simulink model "EHB_MOTOR"  (R2023b)
settings: Solver=FixedStepDiscrete  StartTime=0.0  StopTime=inf  FixedStep=0.0001  RelTol=1e-3  EnableMultiTasking=on
undefined symbols (not defined in the file): CAN_EHB_VCU0x125, CAN_EHB_VCU0x126, CAN_id0x120_Data, Cos_Table, Cos_Table1, EHB_DTC_status, R, Sin_BreakPoint, Sin_BreakPoint1, Sin_Table, Sin_Table1, T
libraries: simulink x30
(part 4 of 9)

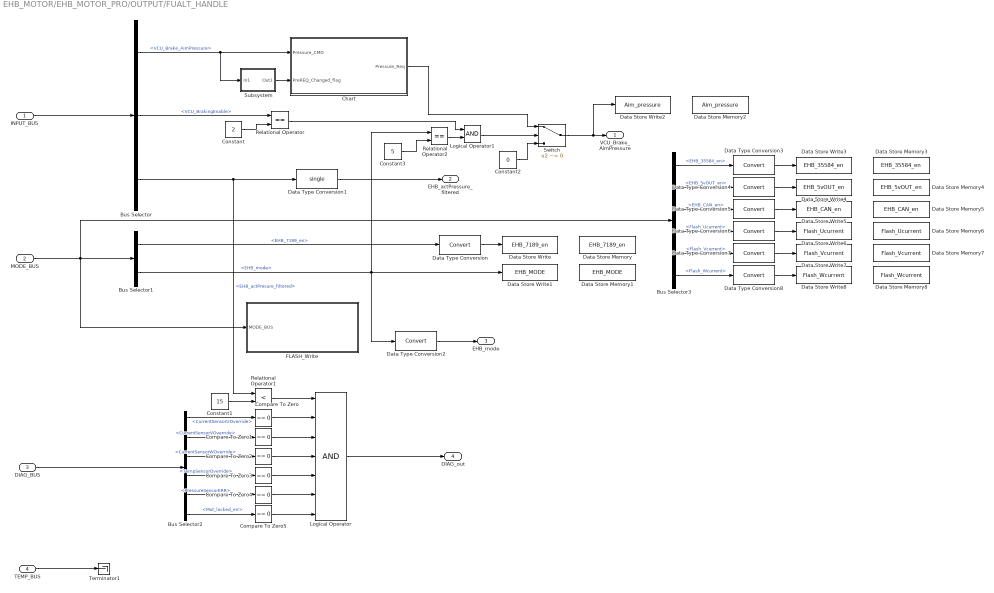
== system EHB_MOTOR/EHB_MOTOR_PRO/OUTPUT/FUALT_HANDLE ==
  INPUT_BUS : Inport
  MODE_BUS : Inport  Port=2
  DIAG_BUS : Inport  Port=3
  TEMP_BUS : Inport  Port=4
  Bus Selector : BusSelector  OutputSignals=CAN_BUS.VCU_Brake_AimPressure,CAN_BUS.VCU_BrakingEnable,AI_BUS.EHB_actPresure_filtered
  Bus Selector1 : BusSelector  OutputSignals=EHB_7189_en,EHB_mode
  Bus Selector2 : BusSelector  OutputSignals=CurrentSensorUOverride,CurrentSensorVOverride,CurrentSensorWOverride,TempSensorOverride,PressureSensorERR,Mot_locked_err
  Bus Selector3 : BusSelector  OutputSignals=EHB_35584_en,EHB_5vOUT_en,EHB_CAN_en,Flash_Ucurrent,Flash_Vcurrent,Flash_Wcurrent
  Chart : Stateflow chart  TreatAsAtomicUnit=on
  Compare To Zero{,1..5} (6 alike) : simulink/Logic and Bit Operations/Compare To Zero  relop===  OutDataTypeStr=boolean
  Constant : Constant  Value=2  OutDataTypeStr=Inherit: Inherit via back propagation
  Constant1 : Constant  Value=15
  Constant2 : Constant  Value=0  OutDataTypeStr=single
  Constant3 : Constant  Value=5  OutDataTypeStr=Inherit: Inherit via back propagation
  Data Store Memory : DataStoreMemory  DataStoreName=EHB_7189_en  ReadBeforeWriteMsg=warning  WriteAfterWriteMsg=warning  WriteAfterReadMsg=warning  ShowAdditionalParam=off  OutDataTypeStr=uint8
  Data Store Memory1 : DataStoreMemory  DataStoreName=EHB_MODE  ReadBeforeWriteMsg=warning  WriteAfterWriteMsg=warning  WriteAfterReadMsg=warning  ShowAdditionalParam=off  OutDataTypeStr=uint8
  Data Store Memory2 : DataStoreMemory  DataStoreName=Aim_pressure  ReadBeforeWriteMsg=warning  WriteAfterWriteMsg=warning  WriteAfterReadMsg=warning  ShowAdditionalParam=off  OutDataTypeStr=single
  Data Store Memory3 : DataStoreMemory  DataStoreName=EHB_35584_en  ReadBeforeWriteMsg=warning  WriteAfterWriteMsg=warning  WriteAfterReadMsg=warning  ShowAdditionalParam=off  OutDataTypeStr=uint8
  Data Store Memory4 : DataStoreMemory  DataStoreName=EHB_5vOUT_en  ReadBeforeWriteMsg=warning  WriteAfterWriteMsg=warning  WriteAfterReadMsg=warning  ShowAdditionalParam=off  OutDataTypeStr=uint8
  Data Store Memory5 : DataStoreMemory  DataStoreName=EHB_CAN_en  ReadBeforeWriteMsg=warning  WriteAfterWriteMsg=warning  WriteAfterReadMsg=warning  ShowAdditionalParam=off  OutDataTypeStr=uint8
  Data Store Memory6 : DataStoreMemory  DataStoreName=Flash_Ucurrent  ReadBeforeWriteMsg=warning  WriteAfterWriteMsg=warning  WriteAfterReadMsg=warning  ShowAdditionalParam=off  OutDataTypeStr=uint16
  Data Store Memory7 : DataStoreMemory  DataStoreName=Flash_Vcurrent  ReadBeforeWriteMsg=warning  WriteAfterWriteMsg=warning  WriteAfterReadMsg=warning  ShowAdditionalParam=off  OutDataTypeStr=uint16
  Data Store Memory8 : DataStoreMemory  DataStoreName=Flash_Wcurrent  ReadBeforeWriteMsg=warning  WriteAfterWriteMsg=warning  WriteAfterReadMsg=warning  ShowAdditionalParam=off  OutDataTypeStr=uint16
  Data Store Write : DataStoreWrite  DataStoreName=EHB_7189_en  DataStoreElements=EHB_7189_en  IndexOptions=Index vector (dialog)  Indices=1  OutputSizes=1
  Data Store Write1 : DataStoreWrite  DataStoreName=EHB_MODE  DataStoreElements=EHB_MODE  IndexOptions=Index vector (dialog)  Indices=1  OutputSizes=1
  Data Store Write2 : DataStoreWrite  DataStoreName=Aim_pressure  DataStoreElements=Aim_pressure  IndexOptions=Index vector (dialog)  Indices=1  OutputSizes=1
  Data Store Write3 : DataStoreWrite  DataStoreName=EHB_35584_en  DataStoreElements=EHB_35584_en  IndexOptions=Index vector (dialog)  Indices=1  OutputSizes=1
  Data Store Write4 : DataStoreWrite  DataStoreName=EHB_5vOUT_en  DataStoreElements=EHB_5vOUT_en  IndexOptions=Index vector (dialog)  Indices=1  OutputSizes=1
  Data Store Write5 : DataStoreWrite  DataStoreName=EHB_CAN_en  DataStoreElements=EHB_CAN_en  IndexOptions=Index vector (dialog)  Indices=1  OutputSizes=1
  Data Store Write6 : DataStoreWrite  DataStoreName=Flash_Ucurrent  DataStoreElements=Flash_Ucurrent  IndexOptions=Index vector (dialog)  Indices=1  OutputSizes=1
  Data Store Write7 : DataStoreWrite  DataStoreName=Flash_Vcurrent  DataStoreElements=Flash_Vcurrent  IndexOptions=Index vector (dialog)  Indices=1  OutputSizes=1
  Data Store Write8 : DataStoreWrite  DataStoreName=Flash_Wcurrent  DataStoreElements=Flash_Wcurrent  IndexOptions=Index vector (dialog)  Indices=1  OutputSizes=1
  Data Type Conversion{,2..8} (8 alike) : DataTypeConversion  SaturateOnIntegerOverflow=off  RndMeth=Floor
  Data Type Conversion1 : DataTypeConversion  OutDataTypeStr=single  SaturateOnIntegerOverflow=off  RndMeth=Floor
  FLASH_Write : Subsystem
  Logical Operator : Logic  Inputs=7  AllPortsSameDT=off  OutDataTypeStr=boolean
  Logical Operator1 : Logic  AllPortsSameDT=off  OutDataTypeStr=boolean
  Relational Operator : RelationalOperator  Operator===  OutDataTypeStr=boolean  RndMeth=Simplest  InputSameDT=off
  Relational Operator1 : RelationalOperator  Operator=<  OutDataTypeStr=boolean  RndMeth=Simplest  InputSameDT=off
  Relational Operator2 : RelationalOperator  Operator===  OutDataTypeStr=boolean  RndMeth=Simplest  InputSameDT=off
  Subsystem : Subsystem
  Switch : Switch  Criteria=u2 ~= 0  SaturateOnIntegerOverflow=off  InputSameDT=off
  Terminator1 : Terminator
  VCU_Brake_AimPressure : Outport  VectorParamsAs1DForOutWhenUnconnected=off
  EHB_actPressure_filtered : Outport  Port=2  VectorParamsAs1DForOutWhenUnconnected=off
  EHB_mode : Outport  Port=3  VectorParamsAs1DForOutWhenUnconnected=off
  DIAG_out : Outport  Port=4  VectorParamsAs1DForOutWhenUnconnected=off
  wires:
  INPUT_BUS/1 -> Bus Selector/1
  Bus Selector/3 -> Data Type Conversion1/1, Relational Operator1/1  "<EHB_actPresure_filtered>"
  TEMP_BUS/1 -> Terminator1/1
  MODE_BUS/1 -> Bus Selector1/1, FLASH_Write/1(MODE_BUS), Bus Selector3/1
  Bus Selector1/1 -> Data Type Conversion/1  "<EHB_7189_en>"
  Data Type Conversion/1 -> Data Store Write/1
  Bus Selector/1 -> Chart/1(Pressure_CMD), Subsystem/1(In1)  "<VCU_Brake_AimPressure>"
  Bus Selector/2 -> Relational Operator/1  "<VCU_BrakingEnable>"
  Constant/1 -> Relational Operator/2
  Relational Operator/1 -> Logical Operator1/1
  Switch/1 -> VCU_Brake_AimPressure/1, Data Store Write2/1
  Constant2/1 -> Switch/3
  Subsystem/1(Out1) -> Chart/2(PreREQ_Changed_flag)
  Chart/1(Pressure_Req) -> Switch/1
  Bus Selector2/4 -> Compare To Zero3/1  "<TempSensorOverride>"
  Bus Selector2/1 -> Compare To Zero/1  "<CurrentSensorUOverride>"
  Compare To Zero/1 -> Logical Operator/2
  Bus Selector2/2 -> Compare To Zero1/1  "<CurrentSensorVOverride>"
  Compare To Zero1/1 -> Logical Operator/3
  Compare To Zero2/1 -> Logical Operator/4
  Compare To Zero3/1 -> Logical Operator/5
  DIAG_BUS/1 -> Bus Selector2/1
  Bus Selector2/3 -> Compare To Zero2/1  "<CurrentSensorWOverride>"
  Logical Operator/1 -> DIAG_out/1
  Constant1/1 -> Relational Operator1/2
  Relational Operator1/1 -> Logical Operator/1
  Bus Selector1/2 -> Data Store Write1/1, Relational Operator2/1, Data Type Conversion2/1  "<EHB_mode>"
  Compare To Zero4/1 -> Logical Operator/6
  Bus Selector2/5 -> Compare To Zero4/1  "<PressureSensorERR>"
  Data Type Conversion1/1 -> EHB_actPressure_filtered/1
  Compare To Zero5/1 -> Logical Operator/7
  Bus Selector2/6 -> Compare To Zero5/1  "<Mot_locked_err>"
  Constant3/1 -> Relational Operator2/2
  Relational Operator2/1 -> Logical Operator1/2
  Logical Operator1/1 -> Switch/2
  Data Type Conversion2/1 -> EHB_mode/1
  Bus Selector3/1 -> Data Type Conversion3/1  "<EHB_35584_en>"
  Data Type Conversion3/1 -> Data Store Write3/1
  Bus Selector3/2 -> Data Type Conversion4/1  "<EHB_5vOUT_en>"
  Data Type Conversion4/1 -> Data Store Write4/1
  Data Type Conversion5/1 -> Data Store Write5/1
  Data Type Conversion6/1 -> Data Store Write6/1
  Bus Selector3/3 -> Data Type Conversion5/1  "<EHB_CAN_en>"
  Bus Selector3/4 -> Data Type Conversion6/1  "<Flash_Ucurrent>"
  Data Type Conversion7/1 -> Data Store Write7/1
  Data Type Conversion8/1 -> Data Store Write8/1
  Bus Selector3/5 -> Data Type Conversion7/1  "<Flash_Vcurrent>"
  Bus Selector3/6 -> Data Type Conversion8/1  "<Flash_Wcurrent>"

== system EHB_MOTOR/EHB_MOTOR_PRO/Pressure_closed/LOWPASS ==
  In1 : Inport
  Add : Sum
  Add1 : Sum  Inputs=+-
  Constant : Constant  Value=0.5  OutDataTypeStr=single
  Constant1 : Constant  OutDataTypeStr=single
  Multiply : Product
  Multiply1 : Product
  Unit Delay : UnitDelay  SampleTime=-1  HasFrameUpgradeWarning=on
  Out1 : Outport  VectorParamsAs1DForOutWhenUnconnected=off
  wires:
  In1/1 -> Multiply/1
  Multiply/1 -> Add/1
  Add/1 -> Unit Delay/1, Out1/1
  Constant/1 -> Add1/2, Multiply/2
  Constant1/1 -> Add1/1
  Add1/1 -> Multiply1/1
  Multiply1/1 -> Add/2
  Unit Delay/1 -> Multiply1/2

== system EHB_MOTOR/EHB_MOTOR_PRO/Speed_closed/Accuracy_Ctrl ==
  Pressure_Cmplt : Inport
  errSpd : Inport  Port=2
  SPDpterm_in : Inport  Port=3
  EHB_Initiate : Inport  Port=4
  Abs : Abs  SaturateOnIntegerOverflow=off
  Constant : Constant  Value=15  OutDataTypeStr=single
  Constant1 : Constant  Value=0  OutDataTypeStr=single
  Logical Operator : Logic  Operator=OR  Inputs=3  AllPortsSameDT=off  OutDataTypeStr=boolean
  Relational Operator : RelationalOperator  Operator=<=  OutDataTypeStr=boolean  RndMeth=Simplest  InputSameDT=off
  Switch : Switch  Criteria=u2 ~= 0  SaturateOnIntegerOverflow=off  InputSameDT=off
  SPDpterm_out : Outport  VectorParamsAs1DForOutWhenUnconnected=off
  wires:
  errSpd/1 -> Abs/1
  Abs/1 -> Relational Operator/1
  Constant/1 -> Relational Operator/2
  Switch/1 -> SPDpterm_out/1
  Constant1/1 -> Switch/1
  SPDpterm_in/1 -> Switch/3
  Relational Operator/1 -> Logical Operator/2
  Pressure_Cmplt/1 -> Logical Operator/1
  Logical Operator/1 -> Switch/2
  EHB_Initiate/1 -> Logical Operator/3

== system EHB_MOTOR/EHB_MOTOR_PRO/Speed_closed/Accuracy_Ctrl1 ==
  Pressure_Cmplt : Inport
  errSpd : Inport  Port=2
  SPDiterm_in : Inport  Port=3
  EHB_Initiate : Inport  Port=4
  Abs : Abs  SaturateOnIntegerOverflow=off
  Constant : Constant  Value=15  OutDataTypeStr=single
  Constant1 : Constant  Value=0  OutDataTypeStr=single
  Logical Operator : Logic  Operator=OR  Inputs=3  AllPortsSameDT=off  OutDataTypeStr=boolean
  Relational Operator : RelationalOperator  Operator=<=  OutDataTypeStr=boolean  RndMeth=Simplest  InputSameDT=off
  Switch : Switch  Criteria=u2 ~= 0  SaturateOnIntegerOverflow=off  InputSameDT=off
  SPDiterm_out : Outport  VectorParamsAs1DForOutWhenUnconnected=off
  wires:
  SPDiterm_in/1 -> Switch/3
  Constant1/1 -> Switch/1
  Switch/1 -> SPDiterm_out/1
  Constant/1 -> Relational Operator/2
  Abs/1 -> Relational Operator/1
  errSpd/1 -> Abs/1
  Relational Operator/1 -> Logical Operator/2
  Logical Operator/1 -> Switch/2
  Pressure_Cmplt/1 -> Logical Operator/1
  EHB_Initiate/1 -> Logical Operator/3

== system EHB_MOTOR/EHB_MOTOR_PRO/Speed_closed/LOWPASS ==
  In1 : Inport
  Add : Sum
  Add1 : Sum  Inputs=+-
  Constant : Constant  Value=0.5  OutDataTypeStr=single
  Constant1 : Constant  OutDataTypeStr=single
  Multiply : Product
  Multiply1 : Product
  Unit Delay : UnitDelay  SampleTime=-1  HasFrameUpgradeWarning=on
  Out1 : Outport  VectorParamsAs1DForOutWhenUnconnected=off
  wires:
  In1/1 -> Multiply/1
  Multiply/1 -> Add/1
  Add/1 -> Unit Delay/1, Out1/1
  Constant/1 -> Add1/2, Multiply/2
  Constant1/1 -> Add1/1
  Add1/1 -> Multiply1/1
  Multiply1/1 -> Add/2
  Unit Delay/1 -> Multiply1/2

== system EHB_MOTOR/EHB_MOTOR_PRO/Speed_closed/WeakMagnetism ==
  note: iq_1
  note: |iq*|cos( △u)
  note: sqrt(Ud*Ud+Uq*Uq)<=Udc/sqrt(3)
  note: id*
  note: id*id+iq*iq<=Ismax*Ismax
  note: iq*
  note: △u
  note: iq*
  note: |iq*|sin( △u)
  Iq_closed_input : Inport
  Speed_desired : Inport  Port=2
  Vd : Inport  Port=3  OutDataTypeStr=single
  Vq : Inport  Port=4  OutDataTypeStr=single
  w_P : Inport  Port=5  OutDataTypeStr=single
  w_I : Inport  Port=6  OutDataTypeStr=single
  -flux/Ld : Saturate  UpperLimit=0  LowerLimit=-76
  1-D Lookup Table : Lookup_n-D  Commented=on  NumberOfTableDimensions=1  BreakpointsForDimension1=[0;2200;2345;2347;2348;2351;2355;2383;2386;2420;2421;2537;2654;2812;3000]  Table=[0;-0.002;-0.07;-0.1;-0.2;-0.3;-0.5;-1;-2;-4;-5;-9;-16;-18;-24]  InternalRulePriority=Speed  RndMeth=Simplest
  Abs : Abs  SaturateOnIntegerOverflow=off
  Add2 : Sum  OutDataTypeStr=single  AccumDataTypeStr=single
  Constant : Constant  Value=0.577  OutDataTypeStr=single
  Constant1 : Constant  Value=0  OutDataTypeStr=single
  Fcn : Fcn  Expr=sqrt(u(1)^2+u(2)^2)/u(3)
  Fcn2 : Fcn  Expr=sqrt(u(1)^2-u(2)^2)
  Gain8 : Gain  Gain=-1
  Ismax : Constant  Value=114  OutDataTypeStr=single  SampleTime=-1
  Mux : Mux  Inputs=3
  Mux2 : Mux  Inputs=2
  Product1 : Product  RndMeth=Zero
  Product2 : Product  RndMeth=Zero
  Saturation : Saturate  UpperLimit=100  LowerLimit=-100  OutDataTypeStr=single
  Saturation Dynamic1 : simulink/Discontinuities/Saturation Dynamic  OutMin=[]  OutMax=[]  OutDataTypeStr=Inherit: Same as second input  OutDataType=fixdt(1, 16)  OutScaling=2^-10  DoSatur=off
  Saturation1 : Saturate  UpperLimit=114  LowerLimit=-114
  Subsystem : Subsystem
  Subsystem2 : Subsystem
  Sum2 : Sum  Inputs=|-+
  Switch : Switch  SaturateOnIntegerOverflow=off  InputSameDT=off
  Terminator : Terminator
  Vdc : Constant  Value=12  OutDataTypeStr=single
  id_desired : Outport
  iq_desired : Outport  Port=2
  wires:
  Subsystem/1(Sin) -> Product1/1
  Constant/1 -> Sum2/2
  Abs/1 -> Product1/2
  -flux/Ld/1 -> Add2/2
  Vq/1 -> Mux/2
  Fcn2/1 -> Gain8/1, Saturation Dynamic1/1
  Gain8/1 -> Saturation Dynamic1/3
  Saturation Dynamic1/1 -> Saturation1/1
  1-D Lookup Table/1 -> Terminator/1
  Ismax/1 -> Mux2/1
  Sum2/1 -> Subsystem2/1(Uerr)
  Fcn/1 -> Sum2/1
  Product1/1 -> -flux/Ld/1
  Vd/1 -> Mux/1
  Saturation/1 -> Mux2/2, id_desired/1
  Subsystem2/1(超前角) -> Subsystem/1(超前角), Switch/2
  Mux2/1 -> Fcn2/1
  Speed_desired/1 -> 1-D Lookup Table/1
  Mux/1 -> Fcn/1
  w_P/1 -> Subsystem2/2(KP)
  Switch/1 -> Saturation Dynamic1/2
  Iq_closed_input/1 -> Product2/1, Abs/1, Switch/1
  Add2/1 -> Saturation/1
  Constant1/1 -> Add2/1
  Product2/1 -> Switch/3
  Subsystem/2(cos) -> Product2/2
  Vdc/1 -> Mux/3
  w_I/1 -> Subsystem2/3(Ki)
  Saturation1/1 -> iq_desired/1

== system EHB_MOTOR/EHB_MOTOR_PRO/Subsystem/CLARK ==
  iA : Inport  OutDataTypeStr=single
  iB : Inport  Port=2  OutDataTypeStr=single
  Add : Sum  OutDataTypeStr=single
  B_Gain : Gain  Gain=2  OutDataTypeStr=single
  Beta_Gain : Gain  Gain=sqrt(3)/3  OutDataTypeStr=single
  alpha_current : Outport  OutDataTypeStr=single  VectorParamsAs1DForOutWhenUnconnected=off
  beta_current : Outport  Port=2  OutDataTypeStr=single  VectorParamsAs1DForOutWhenUnconnected=off
  wires:
  iB/1 -> B_Gain/1
  Beta_Gain/1 -> beta_current/1
  Add/1 -> Beta_Gain/1
  B_Gain/1 -> Add/2
  iA/1 -> Add/1, alpha_current/1

== system EHB_MOTOR/EHB_MOTOR_PRO/Subsystem/Current_PI ==
  id_actual : Inport  OutDataTypeStr=single
  iq_actual : Inport  Port=2  OutDataTypeStr=single
  id_desired : Inport  Port=3  OutDataTypeStr=single
  Iq_desired : Inport  Port=4  OutDataTypeStr=single
  id_P : Inport  Port=5  OutDataTypeStr=single
  id_I : Inport  Port=6  OutDataTypeStr=single
  iq_P : Inport  Port=7  OutDataTypeStr=single
  iq_I : Inport  Port=8  OutDataTypeStr=single
  u_dc : Inport  Port=9
  Pressure_Cmplt : Inport  Port=10
  VCU_Brake_AimPressure : Inport  Port=11
  errPressure : Inport  Port=12
  DIAG : Inport  Port=13
  EHB_Initiate : Inport  Port=14
  EHB_mode : Inport  Port=15
  1-D Lookup Table : Lookup_n-D  NumberOfTableDimensions=1  BreakpointsForDimension1=[-4000,-3000,-2000,-1000,0,1000,2000,3000,4000,5000,6000,7000,8000,9000,10000,11000,12000,13000,14000,15000]  BreakpointsForDimension1DataTypeStr=single  Table=[0.2,0.15,0.1,0.05,0,-0.1,-0.2,-0.24,-0.28,-0.32,-0.36,-0.4,-0.44,-0.48,-0.68,-0.68,-0.68,-0.68,-0.68,-0.68]  TableDataTypeStr=single  ExtrapMethod=Clip  UseLastTableValue=on  InternalRulePriority=Speed  RndMeth=Simplest
  Add1 : Sum  Inputs=+-  OutDataTypeStr=single
  Add2 : Sum  Inputs=+-  OutDataTypeStr=single
  Constant : Constant  Value=0  OutDataTypeStr=single
  Constant1 : Constant  Value=0  OutDataTypeStr=single
  Constant2 : Constant  Value=0  OutDataTypeStr=single
  Id_PI : Subsystem
  Iq_PI : Subsystem
  Logical Operator : Logic  AllPortsSameDT=off  OutDataTypeStr=boolean
  Logical Operator1 : Logic  Operator=NOT  AllPortsSameDT=off  OutDataTypeStr=boolean
  Saturation : Saturate  UpperLimit=0.7  LowerLimit=-0.7  OutDataTypeStr=fixdt(1,16,12)
  Switch : Switch  Criteria=u2 ~= 0  SaturateOnIntegerOverflow=off  InputSameDT=off
  Switch1 : Switch  Criteria=u2 ~= 0  SaturateOnIntegerOverflow=off  InputSameDT=off
  Switch2 : Switch  Criteria=u2 ~= 0  SaturateOnIntegerOverflow=off  InputSameDT=off
  Terminator : Terminator
  Ud : Outport  OutDataTypeStr=single  VectorParamsAs1DForOutWhenUnconnected=off
  Uq : Outport  Port=2  OutDataTypeStr=single  VectorParamsAs1DForOutWhenUnconnected=off
  Ud_out : Outport  Port=3  OutDataTypeStr=single  VectorParamsAs1DForOutWhenUnconnected=off
  Uq_out : Outport  Port=4  OutDataTypeStr=single  VectorParamsAs1DForOutWhenUnconnected=off
  wires:
  Add1/1 -> Id_PI/2(delta_id)
  id_desired/1 -> Add1/1, Id_PI/1(id_desired)
  Add2/1 -> Iq_PI/1(delta_iq)
  Iq_desired/1 -> Add2/1
  iq_actual/1 -> Add2/2
  id_actual/1 -> Add1/2
  Iq_PI/1(pi_out) -> Switch1/1
  id_P/1 -> Id_PI/3(id_P)
  id_I/1 -> Id_PI/4(id_I)
  iq_P/1 -> Iq_PI/2(iq_p)
  iq_I/1 -> Iq_PI/3(iq_I)
  u_dc/1 -> Iq_PI/4(U_dc), Id_PI/5(u_dc)
  Pressure_Cmplt/1 -> Switch2/2, Iq_PI/5(Pressure_Cmplt)
  VCU_Brake_AimPressure/1 -> Iq_PI/6(VCU_Brake_AimPressure)
  errPressure/1 -> 1-D Lookup Table/1
  1-D Lookup Table/1 -> Saturation/1
  Id_PI/1(pi_out) -> Switch2/3
  Switch/1 -> Ud/1
  Switch1/1 -> Uq/1
  Logical Operator/1 -> Switch/2, Switch1/2
  Constant1/1 -> Switch1/3
  Constant/1 -> Switch/3
  Switch2/1 -> Switch/1
  Constant2/1 -> Switch2/1
  DIAG/1 -> Logical Operator/1
  EHB_Initiate/1 -> Logical Operator1/1
  Logical Operator1/1 -> Logical Operator/2
  Saturation/1 -> Terminator/1
  Id_PI/2(Ud_out) -> Ud_out/1
  Iq_PI/2(Uq_out) -> Uq_out/1
  EHB_mode/1 -> Iq_PI/7(EHB_mode)

== system EHB_MOTOR/EHB_MOTOR_PRO/Subsystem/Ia_caculate1 ==
  note: 3#U相2030
      | 8#U相2072
      | 7#U相2007
  Ia_Inte : Inport  OutDataTypeStr=uint16
  Add : Sum  Inputs=+-  OutDataTypeStr=int16
  Data Store Read : DataStoreRead  DataStoreName=Uzero_FOC_adc  DataStoreElements=Uzero_FOC_adc  IndexOptions=Index vector (dialog)  Indices=1  OutputSizes=1
  U_Vot_Cur_coeff : Gain  Gain=0.0814  OutDataTypeStr=single
  Ia_A : Outport  OutDataTypeStr=single  VectorParamsAs1DForOutWhenUnconnected=off
  wires:
  Ia_Inte/1 -> Add/1
  Data Store Read/1 -> Add/2
  Add/1 -> U_Vot_Cur_coeff/1
  U_Vot_Cur_coeff/1 -> Ia_A/1

== system EHB_MOTOR/EHB_MOTOR_PRO/Subsystem/Ib_caculate1 ==
  note: 3#V相2060
      | 8#V相2045
      | 7#V相2013
  Ib_Inte : Inport  OutDataTypeStr=uint16
  Add : Sum  Inputs=+-  OutDataTypeStr=int16
  Constant1 : Constant  Commented=on  Value=4096  OutDataTypeStr=int16
  Data Store Read : DataStoreRead  DataStoreName=Vzero_FOC_adc  DataStoreElements=Vzero_FOC_adc  IndexOptions=Index vector (dialog)  Indices=1  OutputSizes=1
  Divide : Product  Commented=on  Inputs=*/  OutDataTypeStr=single
  Gain : Gain  Commented=on  Gain=33  OutDataTypeStr=int32
  Gain1 : Gain  Commented=on  Gain=0.1  OutDataTypeStr=single
  Gain4 : Gain  Commented=on  Gain=166.67  OutDataTypeStr=int32
  V_Vot_Cur_coeff : Gain  Gain=0.0814  OutDataTypeStr=single
  Ib_A : Outport  OutDataTypeStr=single  VectorParamsAs1DForOutWhenUnconnected=off
  wires:
  Ib_Inte/1 -> Add/1
  Data Store Read/1 -> Add/2
  Constant1/1 -> Divide/2
  Divide/1 -> Gain4/1
  Gain4/1 -> Gain1/1
  Gain/1 -> Divide/1
  Add/1 -> V_Vot_Cur_coeff/1
  V_Vot_Cur_coeff/1 -> Ib_A/1

== system EHB_MOTOR/EHB_MOTOR_PRO/Subsystem/Ic_caculate ==
  note: 3#W相2060
      | 8#W相2033
      | 7#W相2042
  Ic_Inte : Inport  OutDataTypeStr=uint16
  Add : Sum  Inputs=+-  OutDataTypeStr=int16
  Constant1 : Constant  Commented=on  Value=4096  OutDataTypeStr=int16
  Data Store Read : DataStoreRead  DataStoreName=Wzero_FOC_adc  DataStoreElements=Wzero_FOC_adc  IndexOptions=Index vector (dialog)  Indices=1  OutputSizes=1
  Divide : Product  Commented=on  Inputs=*/  OutDataTypeStr=single
  Gain : Gain  Commented=on  Gain=33  OutDataTypeStr=int32
  Gain1 : Gain  Commented=on  Gain=0.1  OutDataTypeStr=single
  Gain4 : Gain  Commented=on  Gain=166.67  OutDataTypeStr=int32
  V_Vot_Cur_coeff : Gain  Gain=0.0814  OutDataTypeStr=single
  Ic_A : Outport  OutDataTypeStr=single  VectorParamsAs1DForOutWhenUnconnected=off
  wires:
  V_Vot_Cur_coeff/1 -> Ic_A/1
  Add/1 -> V_Vot_Cur_coeff/1
  Gain/1 -> Divide/1
  Gain4/1 -> Gain1/1
  Divide/1 -> Gain4/1
  Constant1/1 -> Divide/2
  Data Store Read/1 -> Add/2
  Ic_Inte/1 -> Add/1

== system EHB_MOTOR/EHB_MOTOR_PRO/Subsystem/Inverse_Park_Transform ==
  note: Inverse Park Transform
  Ud : Inport
  Uq : Inport  Port=2
  cos_theta : Inport  Port=3
  sin_theta : Inport  Port=4
  Add : Sum  OutDataTypeStr=single
  Add1 : Sum  Inputs=+-  OutDataTypeStr=single
  Product{,1..3} (4 alike) : Product  OutDataTypeStr=single  RndMeth=Zero
  alpha_voltage : Outport  VectorParamsAs1DForOutWhenUnconnected=off
  beta_voltage : Outport  Port=2  VectorParamsAs1DForOutWhenUnconnected=off
  wires:
  Product/1 -> Add/1
  Product1/1 -> Add/2
  Add/1 -> beta_voltage/1  "beta_voltage"
  Product2/1 -> Add1/1
  Product3/1 -> Add1/2
  Add1/1 -> alpha_voltage/1  "alpha_voltage"
  Ud/1 -> Product/1, Product2/1
  sin_theta/1 -> Product/2, Product3/2
  cos_theta/1 -> Product1/2, Product2/2
  Uq/1 -> Product1/1, Product3/1

== system EHB_MOTOR/EHB_MOTOR_PRO/Subsystem/PWM scaling ==
  PWM_Duty_Time : Inport
  Gain : Gain  Gain=7500  OutDataTypeStr=uint16
  PWM_Numbers : Outport  VectorParamsAs1DForOutWhenUnconnected=off
  wires:
  PWM_Duty_Time/1 -> Gain/1
  Gain/1 -> PWM_Numbers/1

== system EHB_MOTOR/EHB_MOTOR_PRO/Subsystem/Park_Transform ==
  note: Park Transform
  note: Converts balanced two-phase orthogonal stationary system to an orthogonal rotating reference frame.
  alpha : Inport
  beta : Inport  Port=2
  cos_theta : Inport  Port=3
  sin_theta : Inport  Port=4
  Add : Sum  Inputs=-+  OutDataTypeStr=single
  Add1 : Sum  OutDataTypeStr=single
  Product{,1..3} (4 alike) : Product  OutDataTypeStr=single  RndMeth=Zero
  d_current : Outport  OutDataTypeStr=single  VectorParamsAs1DForOutWhenUnconnected=off
  q_current : Outport  Port=2  OutDataTypeStr=single  VectorParamsAs1DForOutWhenUnconnected=off
  wires:
  Product/1 -> Add/1
  Product1/1 -> Add/2
  Add/1 -> q_current/1  "q_current"
  Product2/1 -> Add1/1
  Product3/1 -> Add1/2
  Add1/1 -> d_current/1  "d_current"
  alpha/1 -> Product/1, Product2/1
  beta/1 -> Product3/1, Product1/1
  cos_theta/1 -> Product1/2, Product2/2
  sin_theta/1 -> Product/2, Product3/2

== system EHB_MOTOR/EHB_MOTOR_PRO/Subsystem/SVPWM ==
  Ualfa : Inport  OutDataTypeStr=single
  Ubeta : Inport  Port=2
  Calculate_Phase_Voltages : Subsystem
  Sector Caculate : Subsystem
  phase_voltages : Outport  VectorParamsAs1DForOutWhenUnconnected=off
  N : Outport  Port=2  VectorParamsAs1DForOutWhenUnconnected=off
  wires:
  Ualfa/1 -> Sector Caculate/1(alpha_voltage), Calculate_Phase_Voltages/2(Ualpha)
  Ubeta/1 -> Calculate_Phase_Voltages/3(Ubeta), Sector Caculate/2(beta_voltage)
  Sector Caculate/1(sector) -> Calculate_Phase_Voltages/1(N), N/1
  Calculate_Phase_Voltages/1(phase_voltages) -> phase_voltages/1

== system EHB_MOTOR/EHB_MOTOR_PRO/Subsystem/Subsystem ==
  EHB_mode : Inport
  Theta_Inte : Inport  Port=2
  Theta_zero : Inport  Port=3
  Constant : Constant  Value=3
  Constant1 : Constant  Value=0  OutDataTypeStr=uint16
  Constant2 : Constant  Value=0  OutDataTypeStr=uint16
  Relational Operator : RelationalOperator  Operator===  OutDataTypeStr=boolean  RndMeth=Simplest  InputSameDT=off
  Switch : Switch  Criteria=u2 ~= 0  SaturateOnIntegerOverflow=off  InputSameDT=off
  Switch1 : Switch  Criteria=u2 ~= 0  SaturateOnIntegerOverflow=off  InputSameDT=off
  Theta_Inte_out : Outport  VectorParamsAs1DForOutWhenUnconnected=off
  Theta_zero_out : Outport  Port=2  VectorParamsAs1DForOutWhenUnconnected=off
  wires:
  Constant/1 -> Relational Operator/2
  Theta_Inte/1 -> Switch/3
  Switch/1 -> Theta_Inte_out/1
  Constant1/1 -> Switch/1
  Relational Operator/1 -> Switch/2, Switch1/2
  EHB_mode/1 -> Relational Operator/1
  Theta_zero/1 -> Switch1/3
  Switch1/1 -> Theta_zero_out/1
  Constant2/1 -> Switch1/1

== system EHB_MOTOR/EHB_MOTOR_PRO/Subsystem/Subsystem1 ==
  Ia_A : Inport
  Ib_A : Inport  Port=2
  Ic_A : Inport  Port=3
  N : Inport  Port=4
  Bus Creator : BusCreator  Inputs=3
  Demux : Demux  Outputs=2
  Sector_slect : MultiPortSwitch  Inputs=6  DiagnosticForDefault=None  SaturateOnIntegerOverflow=off  InputSameDT=off
  select1_4 : Subsystem
  select2_5 : Subsystem
  select3_6 : Subsystem
  iA : Outport  VectorParamsAs1DForOutWhenUnconnected=off
  iB : Outport  Port=2  VectorParamsAs1DForOutWhenUnconnected=off
  wires:
  N/1 -> Sector_slect/1
  Ia_A/1 -> Bus Creator/1  "Ia_A"
  Ib_A/1 -> Bus Creator/2  "Ib_A"
  Ic_A/1 -> Bus Creator/3  "Ic_A"
  Bus Creator/1 -> select1_4/1(In1), select2_5/1(In1), select3_6/1(In1)
  Sector_slect/1 -> Demux/1
  Demux/1 -> iA/1
  Demux/2 -> iB/1
  select2_5/1(Out1) -> Sector_slect/6, Sector_slect/3
  select3_6/1(Out1) -> Sector_slect/4, Sector_slect/7
  select1_4/1(Out1) -> Sector_slect/5, Sector_slect/2

== system EHB_MOTOR/EHB_MOTOR_PRO/Subsystem/Subsystem2 ==
  Theta : Inport
  Cos_LookUp : Lookup_n-D  NumberOfTableDimensions=1  BreakpointsForDimension1=Sin_BreakPoint  BreakpointsForDimension3=[5, 7]  BreakpointsForDimension1DataTypeStr=Inherit: Inherit from 'Breakpoint data'  Table=Cos_Table  TableDataTypeStr=Inherit: Inherit from 'Table data'  ExtrapMethod=Clip  InternalRulePriority=Speed  OutDataTypeStr=Inherit: Inherit from 'Table data'  RndMeth=Simplest  InputSameDT=off
  Gain2 : Gain  Gain=7.6699e-04  OutDataTypeStr=single
  Sin_LookUp : Lookup_n-D  NumberOfTableDimensions=1  BreakpointsForDimension1=Sin_BreakPoint  BreakpointsForDimension3=[5, 7]  BreakpointsForDimension1DataTypeStr=Inherit: Inherit from 'Breakpoint data'  Table=Sin_Table  TableDataTypeStr=Inherit: Inherit from 'Table data'  ExtrapMethod=Clip  InternalRulePriority=Speed  OutDataTypeStr=Inherit: Inherit from 'Table data'  RndMeth=Simplest  InputSameDT=off
  Cos : Outport  VectorParamsAs1DForOutWhenUnconnected=off
  Sin : Outport  Port=2  VectorParamsAs1DForOutWhenUnconnected=off
  wires:
  Sin_LookUp/1 -> Sin/1
  Gain2/1 -> Cos_LookUp/1, Sin_LookUp/1
  Theta/1 -> Gain2/1
  Cos_LookUp/1 -> Cos/1

== system EHB_MOTOR/EHB_MOTOR_PRO/Subsystem/System Outputs ==

== system EHB_MOTOR/EHB_MOTOR_PRO/Subsystem/electri_angle zero2 ==
  Theta_Inte : Inport
  Theta_zero : Inport  Port=2  OutDataTypeStr=uint16
  Angle_Val : Switch  Criteria=u2 ~= 0  Threshold=3032  OutDataTypeStr=uint16  SaturateOnIntegerOverflow=off  InputSameDT=off
  Constant : Constant  Value=8191  OutDataTypeStr=uint16
  Max_Count : Constant  Value=32768  OutDataTypeStr=uint16
  Mod : Math  Operator=mod  SignedPower=on
  Relational Operator : RelationalOperator  OutDataTypeStr=boolean  InputSameDT=off
  Theta_to_Max : Sum  Inputs=+-  OutDataTypeStr=uint16
  Zero_to_Theta : Sum  Inputs=++-  OutDataTypeStr=uint16
  Theta : Outport  VectorParamsAs1DForOutWhenUnconnected=off
  wires:
  Max_Count/1 -> Zero_to_Theta/1
  Theta_zero/1 -> Zero_to_Theta/3, Theta_to_Max/2, Relational Operator/2
  Theta_Inte/1 -> Zero_to_Theta/2, Theta_to_Max/1, Relational Operator/1
  Zero_to_Theta/1 -> Angle_Val/3
  Angle_Val/1 -> Mod/1
  Theta_to_Max/1 -> Angle_Val/1
  Relational Operator/1 -> Angle_Val/2
  Mod/1 -> Theta/1
  Constant/1 -> Mod/2

== system EHB_MOTOR/EPB_CTRL/EPB_CTRL/Fault_Handle ==
  In1 : Inport
  Bus Selector : BusSelector  OutputSignals=EPBVoltageLow,EPBVoltageHigh,EPBOverheat,EPBCurrentOverride
  Compare To Zero{,1..3} (4 alike) : simulink/Logic and Bit Operations/Compare To Zero  relop=~=  OutDataTypeStr=boolean
  Logical Operator : Logic  Operator=OR  Inputs=4  AllPortsSameDT=off  OutDataTypeStr=boolean
  Out1 : Outport  VectorParamsAs1DForOutWhenUnconnected=off
  wires:
  In1/1 -> Bus Selector/1
  Bus Selector/1 -> Compare To Zero/1  "<EPBVoltageLow>"
  Bus Selector/2 -> Compare To Zero1/1  "<EPBVoltageHigh>"
  Bus Selector/3 -> Compare To Zero2/1  "<EPBOverheat>"
  Bus Selector/4 -> Compare To Zero3/1  "<EPBCurrentOverride>"
  Compare To Zero/1 -> Logical Operator/1
  Compare To Zero1/1 -> Logical Operator/2
  Compare To Zero2/1 -> Logical Operator/3
  Compare To Zero3/1 -> Logical Operator/4
  Logical Operator/1 -> Out1/1

== system EHB_MOTOR/EPB_CTRL/EPB_Diag/EPBCurrentDiag ==
  note: 200ms
  note: EPB电机电流过流
  EPB1Current : Inport
  EPB2Current : Inport  Port=2
  Chart : Stateflow chart  TreatAsAtomicUnit=on
  Subsystem : Subsystem
  EPBCurrentOverride : Outport  VectorParamsAs1DForOutWhenUnconnected=off
  wires:
  Chart/1(task_200ms()) -> Subsystem/Trigger
  EPB1Current/1 -> Subsystem/1(In1)
  Subsystem/1(Out1) -> EPBCurrentOverride/1
  EPB2Current/1 -> Subsystem/2(In2)

== system EHB_MOTOR/EPB_CTRL/EPB_Diag/EPBOverheatDiag ==
  note: EPB过温故障
  note: 200ms
  EPBTemp : Inport
  Chart : Stateflow chart  TreatAsAtomicUnit=on
  Subsystem1 : Subsystem
  EPBOverheat : Outport  VectorParamsAs1DForOutWhenUnconnected=off
  wires:
  Chart/1(task_200ms()) -> Subsystem1/Trigger
  Subsystem1/1(Out1) -> EPBOverheat/1
  EPBTemp/1 -> Subsystem1/1(In1)

== system EHB_MOTOR/EPB_CTRL/EPB_Diag/EPB_vBATDiag ==
  note: EPB电源电压过低
  note: 200ms
  note: EPB电源电压过高
  EPBVoltage : Inport
  Chart : Stateflow chart  TreatAsAtomicUnit=on
  Subsystem : Subsystem
  EPBVoltageLow : Outport  VectorParamsAs1DForOutWhenUnconnected=off
  EPBVoltageHigh : Outport  Port=2  VectorParamsAs1DForOutWhenUnconnected=off
  wires:
  Subsystem/2(Out2) -> EPBVoltageHigh/1
  Chart/1(task_200ms()) -> Subsystem/Trigger
  Subsystem/1(Out1) -> EPBVoltageLow/1
  EPBVoltage/1 -> Subsystem/1(In1)

== system EHB_MOTOR/EPB_CTRL/Subsystem1/EPB_interface ==
  note: 7181预驱2信号监测（ADC1_AN7）
  note: APB开关信号3(ADC1-AN4)
  note: EPB2温度（ADC1-AN3）
  note: EPB1温度（ADC1_AN2）
  note: EPB2电流（ADC1_AN1）
  note: EPB1电流（ADC1_AN0）
  note: EPB电源监测（ADC0_AN2）
  note: APB开关信号4(ADC1-AN6)
  note: APB开关信号1(ADC1-AN7)
  note: APB开关信号2(ADC1-AN8)
  note: 7181预驱1信号监测（ADC1_AN8）
  EPB_vBAT_AD : Inport
  EPB1_Current_AD : Inport  Port=2
  EPB2_Current_AD : Inport  Port=3
  EPB1_Temp_AD : Inport  Port=4
  EPB2_Temp_AD : Inport  Port=5
  EPB_APBSwitch3_AD : Inport  Port=6
  EPB_APBSwitch4_AD : Inport  Port=7
  EPB_APBSwitch1_AD : Inport  Port=8
  EPB_APBSwitch2_AD : Inport  Port=9
  EPB_7181PreDriver2_AD : Inport  Port=10
  EPB_7181PreDriver1_AD : Inport  Port=11
  12vADC2VOLT : Subsystem
  EPB1DC2Cur : Subsystem
  EPB2DC2Cur : Subsystem
  EPB_7181PreDriver1 : Subsystem
  EPB_7181PreDriver2 : Subsystem
  EPB_APBSwitch1 : Subsystem
  EPB_APBSwitch2 : Subsystem
  EPB_APBSwitch3 : Subsystem
  EPB_APBSwitch4 : Subsystem
  tempADC2Temp : Subsystem
  tempADC2Temp1 : Subsystem
  EPB_vBAT_filtered : Outport  VectorParamsAs1DForOutWhenUnconnected=off
  EPB1_Current_filtered : Outport  Port=2  VectorParamsAs1DForOutWhenUnconnected=off
  EPB2_Current_filtered : Outport  Port=3  VectorParamsAs1DForOutWhenUnconnected=off
  EPB1_Temp : Outport  Port=4  VectorParamsAs1DForOutWhenUnconnected=off
  EPB2_Temp : Outport  Port=5  VectorParamsAs1DForOutWhenUnconnected=off
  EPB_APBSwitch3_filtered : Outport  Port=6  VectorParamsAs1DForOutWhenUnconnected=off
  EPB_APBSwitch4_filtered : Outport  Port=7  VectorParamsAs1DForOutWhenUnconnected=off
  EPB_APBSwitch1_filtered : Outport  Port=8  VectorParamsAs1DForOutWhenUnconnected=off
  EPB_APBSwitch2_filtered : Outport  Port=9  VectorParamsAs1DForOutWhenUnconnected=off
  EPB_7181PreDriver2_filtered : Outport  Port=10  VectorParamsAs1DForOutWhenUnconnected=off
  EPB_7181PreDriver1_filtered : Outport  Port=11  VectorParamsAs1DForOutWhenUnconnected=off
  wires:
  12vADC2VOLT/1(EPB_vBAT_filtered) -> EPB_vBAT_filtered/1
  EPB_vBAT_AD/1 -> 12vADC2VOLT/1(EPB_vBAT_AD)
  EPB1_Current_AD/1 -> EPB1DC2Cur/1(EPB1_Current_AD)
  EPB1DC2Cur/1(EPB1_Current_filtered) -> EPB1_Current_filtered/1
  EPB2DC2Cur/1(EPB2_Current_filtered) -> EPB2_Current_filtered/1
  EPB2_Current_AD/1 -> EPB2DC2Cur/1(EPB2_Current_AD)
  tempADC2Temp/1(EPB1_Temp) -> EPB1_Temp/1
  EPB1_Temp_AD/1 -> tempADC2Temp/1(EPB1_Temp_AD)
  EPB2_Temp_AD/1 -> tempADC2Temp1/1(EPB2_Temp_AD)
  tempADC2Temp1/1(EPB2_Temp) -> EPB2_Temp/1
  EPB_APBSwitch3/1(EPB_APBSwitch3_filtered) -> EPB_APBSwitch3_filtered/1
  EPB_APBSwitch3_AD/1 -> EPB_APBSwitch3/1(EPB_APBSwitch3_AD)
  EPB_APBSwitch4_AD/1 -> EPB_APBSwitch4/1(EPB_APBSwitch4_AD)
  EPB_APBSwitch4/1(EPB_APBSwitch4_filtered) -> EPB_APBSwitch4_filtered/1
  EPB_APBSwitch1/1(EPB_APBSwitch1_filtered) -> EPB_APBSwitch1_filtered/1
  EPB_APBSwitch1_AD/1 -> EPB_APBSwitch1/1(EPB_APBSwitch1_AD)
  EPB_APBSwitch2_AD/1 -> EPB_APBSwitch2/1(EPB_APBSwitch2_AD)
  EPB_APBSwitch2/1(EPB_APBSwitch2_filtered) -> EPB_APBSwitch2_filtered/1
  EPB_7181PreDriver2/1(EPB_7181PreDriver2_filtered) -> EPB_7181PreDriver2_filtered/1
  EPB_7181PreDriver2_AD/1 -> EPB_7181PreDriver2/1(EPB_7181PreDriver2_AD)
  EPB_7181PreDriver1_AD/1 -> EPB_7181PreDriver1/1(EPB_7181PreDriver1_AD)
  EPB_7181PreDriver1/1(EPB_7181PreDriver1_filtered) -> EPB_7181PreDriver1_filtered/1

== system EHB_MOTOR/EHB_MOTOR_PRO/DIAG/5vDiag/Subsystem ==
  note: 当使能5v输出时，无法进行5V输出或输出电压低于4.8V
  note: 4.8V
  In1 : Inport
  function : TriggerPort  TriggerType=function-call  VariantControl=Variant
  Constant : Constant  Value=0  OutDataTypeStr=uint8
  Data Store Memory1 : DataStoreMemory  DataStoreName=V5Voltage_C  ReadBeforeWriteMsg=warning  WriteAfterWriteMsg=warning  WriteAfterReadMsg=warning  ShowAdditionalParam=off  OutDataTypeStr=uint16
  Data Store Memory4 : DataStoreMemory  DataStoreName=V5VoltageMIN_C  ReadBeforeWriteMsg=warning  WriteAfterWriteMsg=warning  WriteAfterReadMsg=warning  ShowAdditionalParam=off  OutDataTypeStr=uint16
  Data Store Read : DataStoreRead  DataStoreName=V5Voltage_C  DataStoreElements=V5Voltage_C  IndexOptions=Index vector (dialog)  Indices=1  OutputSizes=1
  Data Store Read1 : DataStoreRead  DataStoreName=V5VoltageMIN_C  DataStoreElements=V5VoltageMIN_C  IndexOptions=Index vector (dialog)  Indices=1  OutputSizes=1
  ErrorSignalCount1 : Stateflow chart  TreatAsAtomicUnit=on
  Relational Operator : RelationalOperator  Operator=<  OutDataTypeStr=boolean  RndMeth=Simplest  InputSameDT=off
  Out1 : Outport  VectorParamsAs1DForOutWhenUnconnected=off
  wires:
  Constant/1 -> ErrorSignalCount1/3(Recover)
  Data Store Read/1 -> ErrorSignalCount1/2(V5VoltageMIN_C)
  Relational Operator/1 -> ErrorSignalCount1/1(V5Voltage)
  ErrorSignalCount1/1(V5VoltageMIN) -> Out1/1
  In1/1 -> Relational Operator/1
  Data Store Read1/1 -> Relational Operator/2

== system EHB_MOTOR/EHB_MOTOR_PRO/DIAG/AngleSensorDiag/Subsystem ==
  note: 角度信号周期超过[0,32768]
  note: 0
  note: 32768
  In1 : Inport
  function : TriggerPort  TriggerType=function-call  VariantControl=Variant
  Constant : Constant  Value=0  OutDataTypeStr=uint8
  Data Store Memory1 : DataStoreMemory  DataStoreName=AngleSensorSignalOverride_C  ReadBeforeWriteMsg=warning  WriteAfterWriteMsg=warning  WriteAfterReadMsg=warning  ShowAdditionalParam=off  OutDataTypeStr=uint16
  Data Store Memory4 : DataStoreMemory  DataStoreName=AngleSensorSignalMIN_C  ReadBeforeWriteMsg=warning  WriteAfterWriteMsg=warning  WriteAfterReadMsg=warning  ShowAdditionalParam=off  OutDataTypeStr=uint16
  Data Store Memory5 : DataStoreMemory  DataStoreName=AngleSensorSignalMAX_C  ReadBeforeWriteMsg=warning  WriteAfterWriteMsg=warning  WriteAfterReadMsg=warning  ShowAdditionalParam=off  OutDataTypeStr=uint16
  Data Store Read : DataStoreRead  DataStoreName=AngleSensorSignalOverride_C  DataStoreElements=AngleSensorSignalOverride_C  IndexOptions=Index vector (dialog)  Indices=1  OutputSizes=1
  Data Store Read1 : DataStoreRead  DataStoreName=AngleSensorSignalMIN_C  DataStoreElements=AngleSensorSignalMIN_C  IndexOptions=Index vector (dialog)  Indices=1  OutputSizes=1
  Data Store Read2 : DataStoreRead  DataStoreName=AngleSensorSignalMAX_C  DataStoreElements=AngleSensorSignalMAX_C  IndexOptions=Index vector (dialog)  Indices=1  OutputSizes=1
  ErrorSignalCount : Stateflow chart  TreatAsAtomicUnit=on
  Logical Operator : Logic  Operator=OR  AllPortsSameDT=off  OutDataTypeStr=boolean
  Relational Operator : RelationalOperator  Operator=<  OutDataTypeStr=boolean  RndMeth=Simplest  InputSameDT=off
  Relational Operator1 : RelationalOperator  Operator=>  OutDataTypeStr=boolean  RndMeth=Simplest  InputSameDT=off
  Out1 : Outport  VectorParamsAs1DForOutWhenUnconnected=off
  wires:
  Data Store Read1/1 -> Relational Operator/2
  In1/1 -> Relational Operator/1, Relational Operator1/1
  Data Store Read2/1 -> Relational Operator1/2
  ErrorSignalCount/1(AngleSensorSignalOverride) -> Out1/1
  Relational Operator1/1 -> Logical Operator/2
  Relational Operator/1 -> Logical Operator/1
  Logical Operator/1 -> ErrorSignalCount/1(AngleSensorSignal)
  Data Store Read/1 -> ErrorSignalCount/2(AngleSensorSignalOverride_C)
  Constant/1 -> ErrorSignalCount/3(Recover)

== system EHB_MOTOR/EHB_MOTOR_PRO/DIAG/AngleSensorDiag/Subsystem1 ==
  note: 在一定时间内SPI读取5012的值一直为0
  In1 : Inport
  function : TriggerPort  TriggerType=function-call  VariantControl=Variant
  Constant : Constant  Value=0  OutDataTypeStr=uint8
  Constant1 : Constant  Value=0
  Data Store Memory1 : DataStoreMemory  DataStoreName=AngleSensorSignalLost_C  ReadBeforeWriteMsg=warning  WriteAfterWriteMsg=warning  WriteAfterReadMsg=warning  ShowAdditionalParam=off  OutDataTypeStr=uint16
  Data Store Read : DataStoreRead  DataStoreName=AngleSensorSignalLost_C  DataStoreElements=AngleSensorSignalLost_C  IndexOptions=Index vector (dialog)  Indices=1  OutputSizes=1
  ErrorSignalCount : Stateflow chart  TreatAsAtomicUnit=on
  Relational Operator : RelationalOperator  Operator===  OutDataTypeStr=boolean  RndMeth=Simplest  InputSameDT=off
  Out1 : Outport  VectorParamsAs1DForOutWhenUnconnected=off
  wires:
  Constant/1 -> ErrorSignalCount/3(Recover)
  Data Store Read/1 -> ErrorSignalCount/2(AngleSensorSignalLost_C)
  Relational Operator/1 -> ErrorSignalCount/1(AngleSensorSignal)
  ErrorSignalCount/1(AngleSensorSignalLost) -> Out1/1
  In1/1 -> Relational Operator/1
  Constant1/1 -> Relational Operator/2

== system EHB_MOTOR/EHB_MOTOR_PRO/DIAG/AngleSensorDiag/Subsystem2 ==
  note: TBD
  In1 : Inport
  function : TriggerPort  TriggerType=function-call  VariantControl=Variant
  Constant : Constant  Value=0  OutDataTypeStr=uint8
  Constant1 : Constant  Value=0
  Data Store Memory1 : DataStoreMemory  DataStoreName=AngleSensorNoCal_C  ReadBeforeWriteMsg=warning  WriteAfterWriteMsg=warning  WriteAfterReadMsg=warning  ShowAdditionalParam=off  OutDataTypeStr=uint16
  Data Store Read : DataStoreRead  DataStoreName=AngleSensorNoCal_C  DataStoreElements=AngleSensorNoCal_C  IndexOptions=Index vector (dialog)  Indices=1  OutputSizes=1
  ErrorSignalCount : Stateflow chart  TreatAsAtomicUnit=on
  Relational Operator : RelationalOperator  Operator===  OutDataTypeStr=boolean  RndMeth=Simplest  InputSameDT=off
  Out1 : Outport  VectorParamsAs1DForOutWhenUnconnected=off
  wires:
  Constant/1 -> ErrorSignalCount/3(Recover)
  Relational Operator/1 -> ErrorSignalCount/1(AngleSensorSignal)
  In1/1 -> Relational Operator/1
  Data Store Read/1 -> ErrorSignalCount/2(AngleSensorNoCal_C)
  ErrorSignalCount/1(AngleSensorNoCal) -> Out1/1
  Constant1/1 -> Relational Operator/2

== system EHB_MOTOR/EHB_MOTOR_PRO/DIAG/Chip7189Diag/Subsystem ==
  note: 检测到预驱芯片故障引脚出现低电平信号
  In1 : Inport
  function : TriggerPort  TriggerType=function-call  VariantControl=Variant
  Constant : Constant  Value=0
  Constant1 : Constant  Value=0  OutDataTypeStr=uint8
  Data Store Memory1 : DataStoreMemory  DataStoreName=Chip7189Err_C  ReadBeforeWriteMsg=warning  WriteAfterWriteMsg=warning  WriteAfterReadMsg=warning  ShowAdditionalParam=off  OutDataTypeStr=uint16
  Data Store Read2 : DataStoreRead  DataStoreName=Chip7189Err_C  DataStoreElements=Chip7189Err_C  IndexOptions=Index vector (dialog)  Indices=1  OutputSizes=1
  ErrorSignalCount : Stateflow chart  TreatAsAtomicUnit=on
  Relational Operator : RelationalOperator  Operator===  OutDataTypeStr=boolean  RndMeth=Simplest  InputSameDT=off
  Out1 : Outport  VectorParamsAs1DForOutWhenUnconnected=off
  wires:
  Constant1/1 -> ErrorSignalCount/3(Recover)
  In1/1 -> Relational Operator/1
  Constant/1 -> Relational Operator/2
  ErrorSignalCount/1(Chip7189Err) -> Out1/1
  Data Store Read2/1 -> ErrorSignalCount/2(Chip7189Err_C)
  Relational Operator/1 -> ErrorSignalCount/1(Chip7189)

== system EHB_MOTOR/EHB_MOTOR_PRO/DIAG/CurrentSensorDiag/Subsystem ==
  note: 电机未输出时检测的U相电流信号异常
  In1 : Inport
  function : TriggerPort  TriggerType=function-call  VariantControl=Variant
  Abs : Abs  SaturateOnIntegerOverflow=off
  Constant : Constant  Value=0  OutDataTypeStr=uint8
  Data Store Memory1 : DataStoreMemory  DataStoreName=CurrentSensorUOverride_C  ReadBeforeWriteMsg=warning  WriteAfterWriteMsg=warning  WriteAfterReadMsg=warning  ShowAdditionalParam=off  OutDataTypeStr=uint16
  Data Store Memory5 : DataStoreMemory  DataStoreName=CurrentSensorUMAX_C  ReadBeforeWriteMsg=warning  WriteAfterWriteMsg=warning  WriteAfterReadMsg=warning  ShowAdditionalParam=off  OutDataTypeStr=single
  Data Store Read : DataStoreRead  DataStoreName=CurrentSensorUOverride_C  DataStoreElements=CurrentSensorUOverride_C  IndexOptions=Index vector (dialog)  Indices=1  OutputSizes=1
  Data Store Read2 : DataStoreRead  DataStoreName=CurrentSensorUMAX_C  DataStoreElements=CurrentSensorUMAX_C  IndexOptions=Index vector (dialog)  Indices=1  OutputSizes=1
  ErrorSignalCount : Stateflow chart  TreatAsAtomicUnit=on
  Relational Operator1 : RelationalOperator  Operator=>  OutDataTypeStr=boolean  RndMeth=Simplest  InputSameDT=off
  Out1 : Outport  VectorParamsAs1DForOutWhenUnconnected=off
  wires:
  In1/1 -> Abs/1
  Data Store Read2/1 -> Relational Operator1/2
  ErrorSignalCount/1(CurrentSensorUOverride) -> Out1/1
  Relational Operator1/1 -> ErrorSignalCount/1(CurrentSensorU)
  Data Store Read/1 -> ErrorSignalCount/2(CurrentSensorUOverride_C)
  Constant/1 -> ErrorSignalCount/3(Recover)
  Abs/1 -> Relational Operator1/1

== system EHB_MOTOR/EHB_MOTOR_PRO/DIAG/CurrentSensorDiag/Subsystem1 ==
  note: 电机未输出时检测的V相电流信号异常
  In1 : Inport
  function : TriggerPort  TriggerType=function-call  VariantControl=Variant
  Abs : Abs  SaturateOnIntegerOverflow=off
  Constant : Constant  Value=0  OutDataTypeStr=uint8
  Data Store Memory1 : DataStoreMemory  DataStoreName=CurrentSensorVOverride_C  ReadBeforeWriteMsg=warning  WriteAfterWriteMsg=warning  WriteAfterReadMsg=warning  ShowAdditionalParam=off  OutDataTypeStr=uint16
      settings: LockScale=on
  Data Store Memory5 : DataStoreMemory  DataStoreName=CurrentSensorVMAX_C  ReadBeforeWriteMsg=warning  WriteAfterWriteMsg=warning  WriteAfterReadMsg=warning  ShowAdditionalParam=off  OutDataTypeStr=single
  Data Store Read : DataStoreRead  DataStoreName=CurrentSensorVOverride_C  DataStoreElements=CurrentSensorVOverride_C  IndexOptions=Index vector (dialog)  Indices=1  OutputSizes=1
  Data Store Read2 : DataStoreRead  DataStoreName=CurrentSensorVMAX_C  DataStoreElements=CurrentSensorVMAX_C  IndexOptions=Index vector (dialog)  Indices=1  OutputSizes=1
  ErrorSignalCount : Stateflow chart  TreatAsAtomicUnit=on
  Relational Operator1 : RelationalOperator  Operator=>  OutDataTypeStr=boolean  RndMeth=Simplest  InputSameDT=off
  Out1 : Outport  VectorParamsAs1DForOutWhenUnconnected=off
  wires:
  Constant/1 -> ErrorSignalCount/3(Recover)
  Data Store Read/1 -> ErrorSignalCount/2(CurrentSensorVOverride_C)
  Relational Operator1/1 -> ErrorSignalCount/1(CurrentSensorV)
  ErrorSignalCount/1(CurrentSensorVOverride) -> Out1/1
  Data Store Read2/1 -> Relational Operator1/2
  In1/1 -> Abs/1
  Abs/1 -> Relational Operator1/1

== system EHB_MOTOR/EHB_MOTOR_PRO/DIAG/CurrentSensorDiag/Subsystem2 ==
  note: 电机未输出时检测的W相电流信号异常
  In1 : Inport
  function : TriggerPort  TriggerType=function-call  VariantControl=Variant
  Abs : Abs  SaturateOnIntegerOverflow=off
  Constant : Constant  Value=0  OutDataTypeStr=uint8
  Data Store Memory1 : DataStoreMemory  DataStoreName=CurrentSensorWOverride_C  ReadBeforeWriteMsg=warning  WriteAfterWriteMsg=warning  WriteAfterReadMsg=warning  ShowAdditionalParam=off  OutDataTypeStr=uint16
  Data Store Memory5 : DataStoreMemory  DataStoreName=CurrentSensorWMAX_C  ReadBeforeWriteMsg=warning  WriteAfterWriteMsg=warning  WriteAfterReadMsg=warning  ShowAdditionalParam=off  OutDataTypeStr=single
  Data Store Read : DataStoreRead  DataStoreName=CurrentSensorWOverride_C  DataStoreElements=CurrentSensorWOverride_C  IndexOptions=Index vector (dialog)  Indices=1  OutputSizes=1
  Data Store Read2 : DataStoreRead  DataStoreName=CurrentSensorWMAX_C  DataStoreElements=CurrentSensorWMAX_C  IndexOptions=Index vector (dialog)  Indices=1  OutputSizes=1
  ErrorSignalCount : Stateflow chart  TreatAsAtomicUnit=on
  Relational Operator1 : RelationalOperator  Operator=>  OutDataTypeStr=boolean  RndMeth=Simplest  InputSameDT=off
  Out1 : Outport  VectorParamsAs1DForOutWhenUnconnected=off
  wires:
  In1/1 -> Abs/1
  Data Store Read2/1 -> Relational Operator1/2
  ErrorSignalCount/1(CurrentSensorWOverride) -> Out1/1
  Data Store Read/1 -> ErrorSignalCount/2(CurrentSensorWOverride_C)
  Constant/1 -> ErrorSignalCount/3(Recover)
  Abs/1 -> Relational Operator1/1
  Relational Operator1/1 -> ErrorSignalCount/1(CurrentSensorW)
